simulink model "early_return_logic_eg1_1"  (R2018a)
settings: Solver=VariableStepAuto  StartTime=0.0  StopTime=10.0  RelTol=1e-3
settings Model: Creator=86188  LastModifiedBy=86188

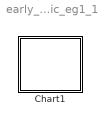
== system early_return_logic_eg1_1 ==
  Chart1 : Stateflow chart  TreatAsAtomicUnit=on

== stateflow chart early_return_logic_eg1_1/Chart1 ==
  settings: executeAtInitialization=1
  state A
  state B
  state C
  (default) -> A
  A -> B [order 1] : [data==1]{data=2;send(F);}
  A -> C [order 2] : F
  data: data local =1
  events: F local FUNCTION_CALL_EVENT
